simulink model "wb_poco_al_intfract_v00"  (Simulink 6.2)
settings: Solver=ode45  StartTime=0.0  StopTime=2^23  RelTol=1e-3
libraries: xbsIndex_r3 x705, xps_library x24, delay_lib x6, fft_library x2, pfb_library x1
(part 1 of 6)
settings Model: LastModifiedBy=sandeep
settings DebuggingCC: SolverPrmCheckMsg=warning

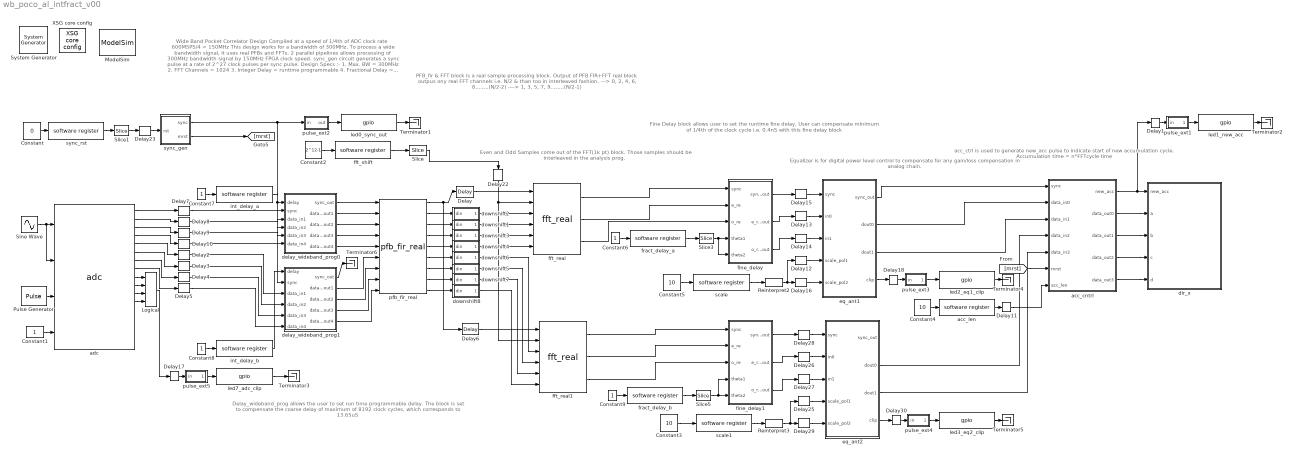
== system wb_poco_al_intfract_v00 ==
  note: Even and Odd Samples come out of the FFT(1k pt) block.
      | Those samples should be interleaved in the analysis prog.
  note: Wide Band Pocket Correlator Design Compiled at a speed of 1/4th of ADC clock rate 600MSPS/4 = 150MHz
      | This design works for a bandwidth of 300MHz. To process a wide bandwidth signal, it uses real PFBs and FFTs.
      | 2 parallel pipelines allows processing of 300MHz bandwidth signal by 150MHz FPGA clock speed.
      | sync_gen circuit generates a sync pulse at a rate of 2^27 clock pulses per sync pulse.
      | Design Specs :-
      | 1. Max. BW = 300MHz
      | 2. FFT Channels = 1024
      | 3. Integer Delay = runtime programmable
      | 4. Fractional Delay = runtime programmable
      | 5. Accumulation time = user cofigurable
  note: PFB_fir & FFT block is a real sample processing block.
      | Output of PFB FIR+FFT real block outpus ony real FFT channels i.e. N/2
      | & than too in interleaved fashion.
      | ---> 0, 2, 4, 6, 8........(N/2-2)
      | ----> 1, 3, 5, 7, 9........(N/2-1)
  note: Equalizer is for digital power level control
      | to compensate for any gain/loss compensation in analog chain.
  note: acc_ctrl is used to generate new_acc pulse
      | to indicate start of new accumulation cycle.
      | Accumulation time = n*FFTcycle time
  note: Delay_wideband_prog allows the user to set run time programmable delay.
      | The block is set to compensate the coarse delay of  maximum of 8192 clock cycles,
      | which corresponds to 13.65uS
  note: Fine Delay block allows user to set the runtime fine delay.
      | User can compensate minimum of 1/4th of the clock cycle i.e. 0.4nS with this fine delay block
  " System Generator" : xbsIndex_r3/ System Generator  Tag=genX  xilinxfamily=Virtex2P  part=xc2vp50  speed=-7  package=ff1152  synthesis_tool=XST  directory=./wb_poco_al_intfract_v00/sysgen  testbench=off  simulink_period=1  sysclk_period=6.6225  incr_netlist=off  trim_vbits=Everywhere in SubSystem  dbl_ovrd=According to Block Masks  core_generation=According to Block Masks  run_coregen=off  deprecated_control=off  eval_field=0
      settings: AttributesFormatString=System\nGenerator
  Constant : Constant  Value=0
  Constant{1,6..9} (5 alike) : Constant
  Constant2 : Constant  Value=2^12-1
  Constant3 : Constant  Value=10
  Constant4 : Constant  Value=10
  Constant5 : Constant  Value=10
  Delay : xbsIndex_r3/Delay  latency=2  reg_retiming=off  explicit_period=off  period=1  en=off  accept_only_valid=off  init_zero=on  dbl_ovrd=off  show_param=off
      settings: xl_area=[0, 0, 0, 0, 0, 0, 0]
  Delay{1,11..18,23,25..30} (16 alike) : xbsIndex_r3/Delay  latency=3  reg_retiming=on  explicit_period=off  period=1  en=off  accept_only_valid=off  init_zero=on  dbl_ovrd=off  show_param=off
      settings: xl_area=[0, 0, 0, 0, 0, 0, 0]
  Delay{2..5,7..10} (8 alike) : xbsIndex_r3/Delay  latency=2  reg_retiming=on  explicit_period=off  period=1  en=off  accept_only_valid=off  init_zero=on  dbl_ovrd=off  show_param=off
      settings: xl_area=[0, 0, 0, 0, 0, 0, 0]
  Delay22 : xbsIndex_r3/Delay  Orientation=down  latency=5  reg_retiming=on  explicit_period=off  period=1  en=off  accept_only_valid=off  init_zero=on  dbl_ovrd=off  show_param=off
      settings: xl_area=[0, 0, 0, 0, 0, 0, 0]
  Delay6 : xbsIndex_r3/Delay  latency=2  reg_retiming=off  explicit_period=off  period=1  en=off  accept_only_valid=off  init_zero=on  dbl_ovrd=off  show_param=off
      settings: xl_area=[0, 0, 0, 0, 0, 0, 0]
  Logical : xbsIndex_r3/Logical  logical_function=OR  inputs=4  precision=Full  arith_type=Unsigned  n_bits=8  bin_pt=2  align_bp=on  latency=0  explicit_period=off  period=1  en=off  dbl_ovrd=off  show_param=off
      settings: xl_area=[0, 0, 0, 0, 0, 0, 0]
  ModelSim : xbsIndex_r3/ModelSim  dir=./modelsim  waveform=on  leave_open=on  skip_compile=off  custom_scripts=off  startup_timeout=40
  Pulse Generator : DiscretePulseGenerator  Period=2^27
  Reinterpret2 : xbsIndex_r3/Reinterpret  force_arith_type=on  arith_type=Unsigned  force_bin_pt=on  bin_pt=3  force_valid=on
  Reinterpret3 : xbsIndex_r3/Reinterpret  force_arith_type=on  arith_type=Unsigned  force_bin_pt=on  bin_pt=3  force_valid=on
  Sine Wave : Sin  SineType=Sample based  Frequency=1/4  Samples=16  SampleTime=0.25
  Slice : xbsIndex_r3/Slice  mode=Upper Bit Location + Width  nbits=12  bit1=0  base1=MSB of Input  bit0=0  base0=LSB of Input  boolean_output=off  explicit_period=off  period=1  dbl_ovrd=off
  Slice1 : xbsIndex_r3/Slice  mode=Lower Bit Location + Width  nbits=1  bit1=0  base1=MSB of Input  bit0=0  base0=LSB of Input  boolean_output=on  explicit_period=off  period=1  dbl_ovrd=off
  Slice3 : xbsIndex_r3/Slice  mode=Lower Bit Location + Width  nbits=8  bit1=0  base1=MSB of Input  bit0=0  base0=LSB of Input  boolean_output=off  explicit_period=off  period=1  dbl_ovrd=off
  Slice5 : xbsIndex_r3/Slice  mode=Lower Bit Location + Width  nbits=8  bit1=0  base1=MSB of Input  bit0=0  base0=LSB of Input  boolean_output=off  explicit_period=off  period=1  dbl_ovrd=off
  Terminator{1..6} (6 alike) : Terminator
  XSG core config : xps_library/XSG core config  Tag=xps:xsg  hw_sys=iBOB  ibob_linux=off  clk_src=adc1_clk  gpio_clk_io_group=iBOB:sma  gpio_clk_bit_index=0  clk_rate=151  sample_period=1  synthesis_tool=XST  mpc_type=powerpc405
  acc_cntrl : Subsystem  mask{chan_bits=8}
      mask prompts: chan_bits "Number of Channels (2^?)"
  acc_len : xps_library/software register  Tag=xps:sw_reg  io_dir=From Processor  arith_type=Unsigned  bitwidth=32  bin_pt=0  sample_period=1  gw_name=wb_poco_al_intfract_v00_acc_len_user_data_out
  adc : xps_library/adc  Tag=xps:adc  adc_brd=iBOB:adc1  adc_clk_rate=601  adc_interleave=off  sample_period=1
  delay_wideband_prog0 : Subsystem
      settings: AttributesFormatString=Min Delay=28
  delay_wideband_prog1 : Subsystem
      settings: AttributesFormatString=Min Delay=28
  dir_x : Subsystem  mask{n_chans=1024}
      mask prompts: n_chans "Number of Channels"
  downshift1 : Subsystem
  downshift2 : Subsystem
  downshift3 : Subsystem
  downshift4 : Subsystem
  downshift5 : Subsystem
  downshift6 : Subsystem
  downshift7 : Subsystem
  downshift8 : Subsystem
  eq_ant1 : Subsystem  mask{n_chans=512}
      mask prompts: n_chans "Number of Channels"
      mask init:
      | chan_bits=ceil(log2(n_chans));
  eq_ant2 : Subsystem  mask{n_chans=512}
      mask prompts: n_chans "Number of Channels"
      mask init:
      | chan_bits=ceil(log2(n_chans));
  fft_real : fft_library/fft_real  FFTSize=10  BitWidth=18  n_inputs=2  quantization="Round  (unbiased: Even Values)"  overflow=Wrap  add_latency=2  mult_latency=3  bram_latency=2
  fft_real1 : fft_library/fft_real  FFTSize=10  BitWidth=18  n_inputs=2  quantization="Round  (unbiased: Even Values)"  overflow=Wrap  add_latency=2  mult_latency=3  bram_latency=2
  fft_shift : xps_library/software register  Tag=xps:sw_reg  io_dir=From Processor  arith_type=Unsigned  bitwidth=32  bin_pt=0  sample_period=1  gw_name=wb_poco_al_intfract_v00_fft_shift_user_data_out
  fine_delay : Subsystem  AncestorBlock=delay_lib/fine_delay  mask{fft_len=1024, fft_bits=18, theta_bits=11, sine_cos_bits=18}
      mask prompts: fft_len "Number Of FFT Channels"; fft_bits "FFT Input Bit Width"; theta_bits "Sine-Cos LUT Input Bitwidth (Determines the resolution of phase)"; sine_cos_bits "Sine-Cos LUT Output Data Width"
      mask init:
      | %fine_delay_init(gcb,...
      |  %   'fft_len',fft_len,...
      |   %  'fft_bits',fft_bits...
      |    % 'theta_bits',theta_bits,...
      |     %'sine_cos_bits',sine_cos_bits)
  fine_delay1 : Subsystem  AncestorBlock=delay_lib/fine_delay  mask{fft_len=1024, fft_bits=18, theta_bits=11, sine_cos_bits=18}
      mask prompts: fft_len "Number Of FFT Channels"; fft_bits "FFT Input Bit Width"; theta_bits "Sine-Cos LUT Input Bitwidth (Determines the resolution of phase)"; sine_cos_bits "Sine-Cos LUT Output Data Width"
      mask init:
      | %fine_delay_init(gcb,...
      |  %   'fft_len',fft_len,...
      |   %  'fft_bits',fft_bits...
      |    % 'theta_bits',theta_bits,...
      |     %'sine_cos_bits',sine_cos_bits)
  fract_delay_a : xps_library/software register  Tag=xps:sw_reg  io_dir=From Processor  arith_type=Unsigned  bitwidth=32  bin_pt=0  sample_period=1  gw_name=wb_poco_al_intfract_v00_fract_delay_a_user_data_out
  fract_delay_b : xps_library/software register  Tag=xps:sw_reg  io_dir=From Processor  arith_type=Unsigned  bitwidth=32  bin_pt=0  sample_period=1  gw_name=wb_poco_al_intfract_v00_fract_delay_b_user_data_out
  int_delay_a : xps_library/software register  Tag=xps:sw_reg  io_dir=From Processor  arith_type=Unsigned  bitwidth=32  bin_pt=0  sample_period=1  gw_name=wb_poco_al_intfract_v00_int_delay_a_user_data_out
  int_delay_b : xps_library/software register  Tag=xps:sw_reg  io_dir=From Processor  arith_type=Unsigned  bitwidth=32  bin_pt=0  sample_period=1  gw_name=wb_poco_al_intfract_v00_int_delay_b_user_data_out
  led0_sync_out : xps_library/gpio  Tag=xps:gpio  io_group=iBOB:led  io_dir=out  arith_type=Boolean  bitwidth=1  bin_pt=0  bit_index=0  sample_period=1  use_single_ended=off  use_ddr=off  reg_iob=on  reg_clk_phase=0  termination=None
  led1_new_acc : xps_library/gpio  Tag=xps:gpio  io_group=iBOB:led  io_dir=out  arith_type=Boolean  bitwidth=1  bin_pt=0  bit_index=1  sample_period=1  use_single_ended=off  use_ddr=off  reg_iob=on  reg_clk_phase=0  termination=None
  led2_eq1_clip : xps_library/gpio  Tag=xps:gpio  io_group=iBOB:led  io_dir=out  arith_type=Boolean  bitwidth=1  bin_pt=0  bit_index=2  sample_period=1  use_single_ended=off  use_ddr=off  reg_iob=on  reg_clk_phase=0  termination=None
  led3_eq2_clip : xps_library/gpio  Tag=xps:gpio  io_group=iBOB:led  io_dir=out  arith_type=Boolean  bitwidth=1  bin_pt=0  bit_index=3  sample_period=1  use_single_ended=off  use_ddr=off  reg_iob=on  reg_clk_phase=0  termination=None
  led7_adc_clip : xps_library/gpio  Tag=xps:gpio  io_group=iBOB:led  io_dir=out  arith_type=Boolean  bitwidth=1  bin_pt=0  bit_index=7  sample_period=1  use_single_ended=off  use_ddr=off  reg_iob=on  reg_clk_phase=0  termination=None
  pfb_fir_real : pfb_library/pfb_fir_real  PFBSize=10  TotalTaps=4  WindowType=hamming  n_inputs=2  MakeBiplex=on  BitWidthIn=8  BitWidthOut=18  CoeffBitWidth=8  CoeffDistMem=off  add_latency=2  mult_latency=3  bram_latency=2  quantization="Round  (unbiased: +/- Inf)"  fwidth=1
      link override pol1_in1_first_tap/sync_delay/Constant: equ=P=C
      link override pol1_in1_first_tap/sync_delay/Constant1: equ=P=C
      link override pol1_in1_first_tap/sync_delay/Constant2: equ=P=C
      link override pol1_in1_first_tap/sync_delay/Constant3: equ=P=C
      link override pol1_in1_tap2/sync_delay/Constant: equ=P=C
      link override pol1_in1_tap2/sync_delay/Constant1: equ=P=C
      link override pol1_in1_tap2/sync_delay/Constant2: equ=P=C
      link override pol1_in1_tap2/sync_delay/Constant3: equ=P=C
      link override pol1_in1_tap3/sync_delay/Constant: equ=P=C
      link override pol1_in1_tap3/sync_delay/Constant1: equ=P=C
      link override pol1_in1_tap3/sync_delay/Constant2: equ=P=C
      link override pol1_in1_tap3/sync_delay/Constant3: equ=P=C
      link override pol1_in2_first_tap/sync_delay/Constant: equ=P=C
      link override pol1_in2_first_tap/sync_delay/Constant1: equ=P=C
      link override pol1_in2_first_tap/sync_delay/Constant2: equ=P=C
      link override pol1_in2_first_tap/sync_delay/Constant3: equ=P=C
      link override pol1_in2_tap2/sync_delay/Constant: equ=P=C
      link override pol1_in2_tap2/sync_delay/Constant1: equ=P=C
      link override pol1_in2_tap2/sync_delay/Constant2: equ=P=C
      link override pol1_in2_tap2/sync_delay/Constant3: equ=P=C
      link override pol1_in2_tap3/sync_delay/Constant: equ=P=C
      link override pol1_in2_tap3/sync_delay/Constant1: equ=P=C
      link override pol1_in2_tap3/sync_delay/Constant2: equ=P=C
      link override pol1_in2_tap3/sync_delay/Constant3: equ=P=C
      link override pol1_in3_first_tap/sync_delay/Constant: equ=P=C
      link override pol1_in3_first_tap/sync_delay/Constant1: equ=P=C
      link override pol1_in3_first_tap/sync_delay/Constant2: equ=P=C
      link override pol1_in3_first_tap/sync_delay/Constant3: equ=P=C
      link override pol1_in3_tap2/sync_delay/Constant: equ=P=C
      link override pol1_in3_tap2/sync_delay/Constant1: equ=P=C
      link override pol1_in3_tap2/sync_delay/Constant2: equ=P=C
      link override pol1_in3_tap2/sync_delay/Constant3: equ=P=C
      link override pol1_in3_tap3/sync_delay/Constant: equ=P=C
      link override pol1_in3_tap3/sync_delay/Constant1: equ=P=C
      link override pol1_in3_tap3/sync_delay/Constant2: equ=P=C
      link override pol1_in3_tap3/sync_delay/Constant3: equ=P=C
      link override pol1_in4_first_tap/sync_delay/Constant: equ=P=C
      link override pol1_in4_first_tap/sync_delay/Constant1: equ=P=C
      link override pol1_in4_first_tap/sync_delay/Constant2: equ=P=C
      link override pol1_in4_first_tap/sync_delay/Constant3: equ=P=C
      link override pol1_in4_tap2/sync_delay/Constant: equ=P=C
      link override pol1_in4_tap2/sync_delay/Constant1: equ=P=C
      link override pol1_in4_tap2/sync_delay/Constant2: equ=P=C
      link override pol1_in4_tap2/sync_delay/Constant3: equ=P=C
      link override pol1_in4_tap3/sync_delay/Constant: equ=P=C
      link override pol1_in4_tap3/sync_delay/Constant1: equ=P=C
      link override pol1_in4_tap3/sync_delay/Constant2: equ=P=C
      link override pol1_in4_tap3/sync_delay/Constant3: equ=P=C
      link override pol2_in1_first_tap/sync_delay/Constant: equ=P=C
      link override pol2_in1_first_tap/sync_delay/Constant1: equ=P=C
      link override pol2_in1_first_tap/sync_delay/Constant2: equ=P=C
      link override pol2_in1_first_tap/sync_delay/Constant3: equ=P=C
      link override pol2_in1_tap2/sync_delay/Constant: equ=P=C
      link override pol2_in1_tap2/sync_delay/Constant1: equ=P=C
      link override pol2_in1_tap2/sync_delay/Constant2: equ=P=C
      link override pol2_in1_tap2/sync_delay/Constant3: equ=P=C
      link override pol2_in1_tap3/sync_delay/Constant: equ=P=C
      link override pol2_in1_tap3/sync_delay/Constant1: equ=P=C
      link override pol2_in1_tap3/sync_delay/Constant2: equ=P=C
      link override pol2_in1_tap3/sync_delay/Constant3: equ=P=C
      link override pol2_in2_first_tap/sync_delay/Constant: equ=P=C
      link override pol2_in2_first_tap/sync_delay/Constant1: equ=P=C
      link override pol2_in2_first_tap/sync_delay/Constant2: equ=P=C
      link override pol2_in2_first_tap/sync_delay/Constant3: equ=P=C
      link override pol2_in2_tap2/sync_delay/Constant: equ=P=C
      link override pol2_in2_tap2/sync_delay/Constant1: equ=P=C
      link override pol2_in2_tap2/sync_delay/Constant2: equ=P=C
      link override pol2_in2_tap2/sync_delay/Constant3: equ=P=C
      link override pol2_in2_tap3/sync_delay/Constant: equ=P=C
      link override pol2_in2_tap3/sync_delay/Constant1: equ=P=C
      link override pol2_in2_tap3/sync_delay/Constant2: equ=P=C
      link override pol2_in2_tap3/sync_delay/Constant3: equ=P=C
      link override pol2_in3_first_tap/sync_delay/Constant: equ=P=C
      link override pol2_in3_first_tap/sync_delay/Constant1: equ=P=C
      link override pol2_in3_first_tap/sync_delay/Constant2: equ=P=C
      link override pol2_in3_first_tap/sync_delay/Constant3: equ=P=C
      link override pol2_in3_tap2/sync_delay/Constant: equ=P=C
      link override pol2_in3_tap2/sync_delay/Constant1: equ=P=C
      link override pol2_in3_tap2/sync_delay/Constant2: equ=P=C
      link override pol2_in3_tap2/sync_delay/Constant3: equ=P=C
      link override pol2_in3_tap3/sync_delay/Constant: equ=P=C
      link override pol2_in3_tap3/sync_delay/Constant1: equ=P=C
      link override pol2_in3_tap3/sync_delay/Constant2: equ=P=C
      link override pol2_in3_tap3/sync_delay/Constant3: equ=P=C
      link override pol2_in4_first_tap/sync_delay/Constant: equ=P=C
      link override pol2_in4_first_tap/sync_delay/Constant1: equ=P=C
      link override pol2_in4_first_tap/sync_delay/Constant2: equ=P=C
      link override pol2_in4_first_tap/sync_delay/Constant3: equ=P=C
      link override pol2_in4_tap2/sync_delay/Constant: equ=P=C
      link override pol2_in4_tap2/sync_delay/Constant1: equ=P=C
      link override pol2_in4_tap2/sync_delay/Constant2: equ=P=C
      link override pol2_in4_tap2/sync_delay/Constant3: equ=P=C
      link override pol2_in4_tap3/sync_delay/Constant: equ=P=C
      link override pol2_in4_tap3/sync_delay/Constant1: equ=P=C
      link override pol2_in4_tap3/sync_delay/Constant2: equ=P=C
      link override pol2_in4_tap3/sync_delay/Constant3: equ=P=C
  pulse_ext1 : Subsystem  mask{pulse_len=2^23}
      mask prompts: pulse_len "Length of Pulse"
      mask init:
      | bits = ceil(log2(pulse_len+1));
  pulse_ext2 : Subsystem  mask{pulse_len=2^23}
      mask prompts: pulse_len "Length of Pulse"
      mask init:
      | bits = ceil(log2(pulse_len+1));
  pulse_ext3 : Subsystem  mask{pulse_len=2^23}
      mask prompts: pulse_len "Length of Pulse"
      mask init:
      | bits = ceil(log2(pulse_len+1));
  pulse_ext4 : Subsystem  mask{pulse_len=2^23}
      mask prompts: pulse_len "Length of Pulse"
      mask init:
      | bits = ceil(log2(pulse_len+1));
  pulse_ext5 : Subsystem  mask{pulse_len=2^23}
      mask prompts: pulse_len "Length of Pulse"
      mask init:
      | bits = ceil(log2(pulse_len+1));
  scale : xps_library/software register  Tag=xps:sw_reg  io_dir=From Processor  arith_type=Unsigned  bitwidth=32  bin_pt=0  sample_period=1  gw_name=wb_poco_al_intfract_v00_scale_user_data_out
  scale1 : xps_library/software register  Tag=xps:sw_reg  io_dir=From Processor  arith_type=Unsigned  bitwidth=32  bin_pt=0  sample_period=1  gw_name=wb_poco_al_intfract_v00_scale1_user_data_out
  sync_gen : Subsystem  mask{sync_bits=27}
      mask prompts: sync_bits "Sync Period (2^?)"
  sync_rst : xps_library/software register  Tag=xps:sw_reg  io_dir=From Processor  arith_type=Unsigned  bitwidth=32  bin_pt=0  sample_period=1  gw_name=wb_poco_al_intfract_v00_sync_rst_user_data_out
  wires:
  Sine Wave/1 -> adc/1, adc/2
  sync_gen/1(sync) -> pulse_ext2/1(in), delay_wideband_prog0/2(sync), delay_wideband_prog1/2(sync)
  sync_gen/2(mrst) -> [mrst]
  Constant/1 -> sync_rst/1
  sync_rst/1 -> Slice1/1
  Slice1/1 -> Delay23/1
  led0_sync_out/1 -> Terminator1/1
  Pulse Generator/1 -> adc/3
  Constant1/1 -> adc/4
  adc/1 -> Delay7/1
  adc/2 -> Delay8/1
  adc/3 -> Delay9/1
  adc/4 -> Delay10/1
  pfb_fir_real/1 -> Delay/1, Delay6/1
  Constant2/1 -> fft_shift/1
  fft_shift/1 -> Slice/1
  Delay/1 -> fft_real/1
  pfb_fir_real/2 -> downshift2/1(din)
  pfb_fir_real/3 -> downshift1/1(din)
  pfb_fir_real/4 -> downshift3/1(din)
  pfb_fir_real/5 -> downshift4/1(din)
  Slice/1 -> Delay22/1
  downshift2/1(dout) -> fft_real/3
  downshift1/1(dout) -> fft_real/4
  downshift3/1(dout) -> fft_real/5
  downshift4/1(dout) -> fft_real/6
  Delay13/1 -> eq_ant1/2(in0)
  Delay14/1 -> eq_ant1/3(in1)
  Delay15/1 -> eq_ant1/1(sync)
  pulse_ext2/1(out) -> led0_sync_out/1
  pulse_ext3/1(out) -> led2_eq1_clip/1
  eq_ant1/4(clip) -> Delay18/1
  Constant5/1 -> scale/1
  scale/1 -> Reinterpret2/1
  Delay12/1 -> eq_ant1/4(scale_pol1)
  Delay16/1 -> eq_ant1/5(scale_pol2)
  Delay18/1 -> pulse_ext3/1(in)
  Delay22/1 -> fft_real/2, fft_real1/2
  Delay23/1 -> sync_gen/1(rst)
  Reinterpret2/1 -> Delay12/1, Delay16/1
  adc/5 -> Delay2/1
  adc/6 -> Delay3/1
  adc/7 -> Delay4/1
  adc/8 -> Delay5/1
  Delay6/1 -> fft_real1/1
  downshift6/1(dout) -> fft_real1/3
  downshift5/1(dout) -> fft_real1/4
  downshift7/1(dout) -> fft_real1/5
  downshift8/1(dout) -> fft_real1/6
  pfb_fir_real/6 -> downshift6/1(din)
  pfb_fir_real/7 -> downshift5/1(din)
  pfb_fir_real/8 -> downshift7/1(din)
  pfb_fir_real/9 -> downshift8/1(din)
  Delay26/1 -> eq_ant2/2(in0)
  Delay27/1 -> eq_ant2/3(in1)
  Delay28/1 -> eq_ant2/1(sync)
  pulse_ext4/1(out) -> led3_eq2_clip/1
  eq_ant2/4(clip) -> Delay30/1
  Delay25/1 -> eq_ant2/4(scale_pol1)
  Delay29/1 -> eq_ant2/5(scale_pol2)
  Delay30/1 -> pulse_ext4/1(in)
  Constant3/1 -> scale1/1
  scale1/1 -> Reinterpret3/1
  Reinterpret3/1 -> Delay29/1, Delay25/1
  led2_eq1_clip/1 -> Terminator4/1
  led3_eq2_clip/1 -> Terminator5/1
  Constant4/1 -> acc_len/1
  acc_len/1 -> Delay11/1
  Delay11/1 -> acc_cntrl/7(acc_len)
  [mrst] -> acc_cntrl/6(mrst)
  eq_ant1/1(sync_out) -> acc_cntrl/1(sync)
  eq_ant1/2(dout0) -> acc_cntrl/2(data_in0)
  eq_ant1/3(dout1) -> acc_cntrl/3(data_in1)
  eq_ant2/2(dout0) -> acc_cntrl/4(data_in2)
  eq_ant2/3(dout1) -> acc_cntrl/5(data_in3)
  acc_cntrl/1(new_acc) -> dir_x/1(new_acc), Delay1/1
  acc_cntrl/2(data_out0) -> dir_x/2(a)
  acc_cntrl/3(data_out1) -> dir_x/3(b)
  acc_cntrl/4(data_out2) -> dir_x/4(c)
  acc_cntrl/5(data_out3) -> dir_x/5(d)
  pulse_ext1/1(out) -> led1_new_acc/1
  Delay1/1 -> pulse_ext1/1(in)
  led1_new_acc/1 -> Terminator2/1
  pulse_ext5/1(out) -> led7_adc_clip/1
  Delay17/1 -> pulse_ext5/1(in)
  led7_adc_clip/1 -> Terminator3/1
  adc/9 -> Logical/1
  adc/10 -> Logical/2
  adc/11 -> Logical/3
  adc/12 -> Logical/4
  Logical/1 -> Delay17/1
  int_delay_a/1 -> delay_wideband_prog0/1(delay)
  int_delay_b/1 -> delay_wideband_prog1/1(delay)
  Constant7/1 -> int_delay_a/1
  Constant8/1 -> int_delay_b/1
  delay_wideband_prog0/1(sync_out) -> pfb_fir_real/1
  delay_wideband_prog0/2(data_out1) -> pfb_fir_real/2
  delay_wideband_prog0/3(data_out2) -> pfb_fir_real/3
  delay_wideband_prog0/4(data_out3) -> pfb_fir_real/4
  delay_wideband_prog0/5(data_out4) -> pfb_fir_real/5
  Delay7/1 -> delay_wideband_prog0/3(data_in1)
  Delay8/1 -> delay_wideband_prog0/4(data_in2)
  Delay9/1 -> delay_wideband_prog0/5(data_in3)
  Delay10/1 -> delay_wideband_prog0/6(data_in4)
  delay_wideband_prog1/1(sync_out) -> Terminator6/1
  Delay2/1 -> delay_wideband_prog1/3(data_in1)
  Delay3/1 -> delay_wideband_prog1/4(data_in2)
  Delay4/1 -> delay_wideband_prog1/5(data_in3)
  Delay5/1 -> delay_wideband_prog1/6(data_in4)
  delay_wideband_prog1/2(data_out1) -> pfb_fir_real/6
  delay_wideband_prog1/3(data_out2) -> pfb_fir_real/7
  delay_wideband_prog1/4(data_out3) -> pfb_fir_real/8
  delay_wideband_prog1/5(data_out4) -> pfb_fir_real/9
  Constant6/1 -> fract_delay_a/1
  fract_delay_a/1 -> Slice3/1
  Slice3/1 -> fine_delay/4(theta1), fine_delay/5(theta2)
  fft_real/1 -> fine_delay/1(sync)
  fft_real/2 -> fine_delay/2(e_re)
  fft_real/3 -> fine_delay/3(o_re)
  Constant9/1 -> fract_delay_b/1
  fract_delay_b/1 -> Slice5/1
  fine_delay/1(sync_out) -> Delay15/1
  fine_delay/2(e_re_out) -> Delay13/1
  fine_delay/3(o_re_out) -> Delay14/1
  fine_delay1/1(sync_out) -> Delay28/1
  fine_delay1/2(e_re_out) -> Delay26/1
  fine_delay1/3(o_re_out) -> Delay27/1
  Slice5/1 -> fine_delay1/5(theta2), fine_delay1/4(theta1)
  fft_real1/1 -> fine_delay1/1(sync)
  fft_real1/2 -> fine_delay1/2(e_re)
  fft_real1/3 -> fine_delay1/3(o_re)

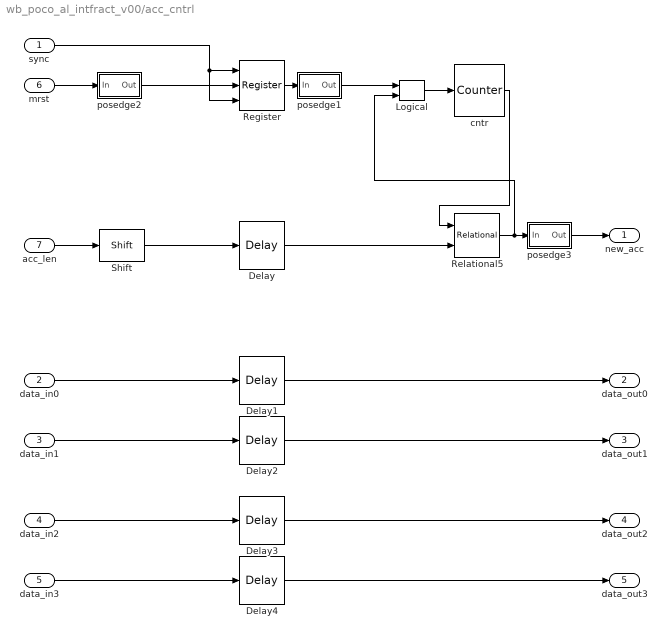
== system wb_poco_al_intfract_v00/acc_cntrl ==
  sync : Inport  Port=1  LatchInput=off
  data_in0 : Inport  Port=2  LatchInput=off
  data_in1 : Inport  Port=3  LatchInput=off
  data_in2 : Inport  Port=4  LatchInput=off
  data_in3 : Inport  Port=5  LatchInput=off
  mrst : Inport  Port=6  LatchInput=off
  acc_len : Inport  Port=7  LatchInput=off
  Delay{,1..4} (5 alike) : xbsIndex_r3/Delay  latency=1  reg_retiming=on  explicit_period=off  period=1  en=off  accept_only_valid=off  init_zero=on  dbl_ovrd=off  show_param=off
      settings: xl_area=[0, 0, 0, 0, 0, 0, 0]
  Logical : xbsIndex_r3/Logical  logical_function=OR  inputs=2  precision=Full  arith_type=Unsigned  n_bits=8  bin_pt=2  align_bp=on  latency=0  explicit_period=off  period=1  en=off  dbl_ovrd=off  show_param=off
      settings: xl_area=[0, 0, 0, 0, 0, 0, 0]
  Register : xbsIndex_r3/Register  init=0  reg_only_valid=off  explicit_period=off  period=1  rst=on  en=on  out_en=off  dbl_ovrd=off  show_param=off
      settings: xl_area=[0, 0, 0, 0, 0, 0, 0]
  Relational5 : xbsIndex_r3/Relational  mode=a>=b  latency=0  explicit_period=on  period=1  en=off  dbl_ovrd=off  show_param=off
      settings: xl_area=[0, 0, 0, 0, 0, 0, 0]
  Shift : xbsIndex_r3/Shift  shift_dir=Left  shift_bits=chan_bits  precision=Full  arith_type="Signed  (2's comp)"  n_bits=8  bin_pt=2  quantization=Truncate  overflow=Wrap  latency=0  explicit_period=off  period=1  en=off  dbl_ovrd=off  show_param=off
      settings: xl_area=[0, 0, 0, 0, 0, 0, 0]
  cntr : xbsIndex_r3/Counter  cnt_type=Free Running  n_bits=32  bin_pt=0  arith_type=Unsigned  start_count=1  cnt_to=Inf  cnt_by_val=1  operation=Up  explicit_period=on  period=1  load_pin=off  rst=on  en=off  dbl_ovrd=off  show_param=off  use_rpm=on  gen_core=off
      settings: xl_area=[0, 0, 0, 0, 0, 0, 0]
  posedge1 : Subsystem  Tag=Rising Edge Detector
  posedge2 : Subsystem  Tag=Rising Edge Detector
  posedge3 : Subsystem  Tag=Rising Edge Detector
  new_acc : Outport
  data_out0 : Outport  Port=2
  data_out1 : Outport  Port=3
  data_out2 : Outport  Port=4
  data_out3 : Outport  Port=5
  wires:
  Relational5/1 -> Logical/2, posedge3/1(In)
  acc_len/1 -> Shift/1
  data_in0/1 -> Delay1/1
  posedge3/1(Out) -> new_acc/1
  Logical/1 -> cntr/1
  Register/1 -> posedge1/1(In)
  posedge2/1(Out) -> Register/2
  posedge1/1(Out) -> Logical/1
  Delay/1 -> Relational5/2
  Delay1/1 -> data_out0/1
  Shift/1 -> Delay/1
  cntr/1 -> Relational5/1
  mrst/1 -> posedge2/1(In)
  sync/1 -> Register/1, Register/3
  data_in1/1 -> Delay2/1
  Delay2/1 -> data_out1/1
  data_in2/1 -> Delay3/1
  Delay3/1 -> data_out2/1
  data_in3/1 -> Delay4/1
  Delay4/1 -> data_out3/1

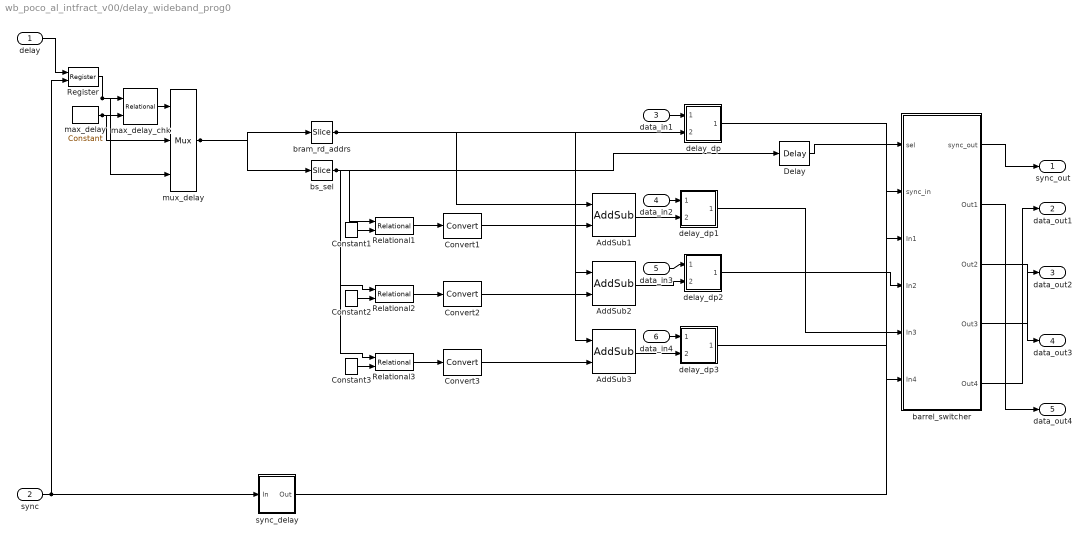
== system wb_poco_al_intfract_v00/delay_wideband_prog0 ==
  delay : Inport  Port=1  LatchInput=off
  sync : Inport  Port=2  LatchInput=off
  data_in1 : Inport  Port=3  LatchInput=off
  data_in2 : Inport  Port=4  LatchInput=off
  data_in3 : Inport  Port=5  LatchInput=off
  data_in4 : Inport  Port=6  LatchInput=off
  AddSub1 : xbsIndex_r3/AddSub  mode=Addition  precision=Full  arith_type=Unsigned  n_bits=11  bin_pt=0  quantization=Truncate  overflow=Wrap  latency=0  explicit_period=off  period=1  use_carryin=off  use_carryout=off  en=off  dbl_ovrd=off  show_param=off  use_core=on  pipeline=off  use_rpm=on  gen_core=off
      settings: xl_area=[0, 0, 0, 0, 0, 0, 0]
  AddSub2 : xbsIndex_r3/AddSub  mode=Addition  precision=Full  arith_type=Unsigned  n_bits=11  bin_pt=0  quantization=Truncate  overflow=Wrap  latency=0  explicit_period=off  period=1  use_carryin=off  use_carryout=off  en=off  dbl_ovrd=off  show_param=off  use_core=on  pipeline=off  use_rpm=on  gen_core=off
      settings: xl_area=[0, 0, 0, 0, 0, 0, 0]
  AddSub3 : xbsIndex_r3/AddSub  mode=Addition  precision=Full  arith_type=Unsigned  n_bits=11  bin_pt=0  quantization=Truncate  overflow=Wrap  latency=0  explicit_period=off  period=1  use_carryin=off  use_carryout=off  en=off  dbl_ovrd=off  show_param=off  use_core=on  pipeline=off  use_rpm=on  gen_core=off
      settings: xl_area=[0, 0, 0, 0, 0, 0, 0]
  Constant1 : xbsIndex_r3/Constant  const=2  equ=P=C  arith_type=Unsigned  n_bits=2  bin_pt=0  opselect=C  inp2=PCIN>>17  opr=+  inp1=P  carry=CIN  iostate=0  explicit_period=on  period=1  dbl_ovrd=off
  Constant2 : xbsIndex_r3/Constant  const=1  equ=P=C  arith_type=Unsigned  n_bits=2  bin_pt=0  opselect=C  inp2=PCIN>>17  opr=+  inp1=P  carry=CIN  iostate=0  explicit_period=on  period=1  dbl_ovrd=off
  Constant3 : xbsIndex_r3/Constant  const=0  equ=P=C  arith_type=Unsigned  n_bits=2  bin_pt=0  opselect=C  inp2=PCIN>>17  opr=+  inp1=P  carry=CIN  iostate=0  explicit_period=on  period=1  dbl_ovrd=off
  Convert1 : xbsIndex_r3/Convert  arith_type=Unsigned  n_bits=1  bin_pt=0  quantization=Truncate  overflow=Wrap  latency=0  explicit_period=off  period=1  dbl_ovrd=off  show_param=off  inserted_by_tool=off  pipeline=off
      settings: xl_area=[0, 0, 0, 0, 0, 0, 0]
  Convert2 : xbsIndex_r3/Convert  arith_type=Unsigned  n_bits=1  bin_pt=0  quantization=Truncate  overflow=Wrap  latency=0  explicit_period=off  period=1  dbl_ovrd=off  show_param=off  inserted_by_tool=off  pipeline=off
      settings: xl_area=[0, 0, 0, 0, 0, 0, 0]
  Convert3 : xbsIndex_r3/Convert  arith_type=Unsigned  n_bits=1  bin_pt=0  quantization=Truncate  overflow=Wrap  latency=0  explicit_period=off  period=1  dbl_ovrd=off  show_param=off  inserted_by_tool=off  pipeline=off
      settings: xl_area=[0, 0, 0, 0, 0, 0, 0]
  Delay : xbsIndex_r3/Delay  latency=5  reg_retiming=off  explicit_period=off  period=1  en=off  accept_only_valid=off  init_zero=on  dbl_ovrd=off  show_param=off
      settings: xl_area=[0, 0, 0, 0, 0, 0, 0]
  Register : xbsIndex_r3/Register  init=0  reg_only_valid=off  explicit_period=off  period=1  rst=off  en=on  out_en=off  dbl_ovrd=off  show_param=off
      settings: xl_area=[0, 0, 0, 0, 0, 0, 0]
  Relational1 : xbsIndex_r3/Relational  mode=a>b  latency=0  explicit_period=off  period=1  en=off  dbl_ovrd=off  show_param=off
      settings: xl_area=[0, 0, 0, 0, 0, 0, 0]
  Relational2 : xbsIndex_r3/Relational  mode=a>b  latency=0  explicit_period=off  period=1  en=off  dbl_ovrd=off  show_param=off
      settings: xl_area=[0, 0, 0, 0, 0, 0, 0]
  Relational3 : xbsIndex_r3/Relational  mode=a>b  latency=0  explicit_period=off  period=1  en=off  dbl_ovrd=off  show_param=off
      settings: xl_area=[0, 0, 0, 0, 0, 0, 0]
  barrel_switcher : Subsystem
      settings: AttributesFormatString=n_inputs=2
  bram_rd_addrs : xbsIndex_r3/Slice  mode=Lower Bit Location + Width  nbits=11  bit1=0  base1=MSB of Input  bit0=2  base0=LSB of Input  boolean_output=off  explicit_period=off  period=1  dbl_ovrd=off
  bs_sel : xbsIndex_r3/Slice  mode=Lower Bit Location + Width  nbits=2  bit1=0  base1=MSB of Input  bit0=0  base0=LSB of Input  boolean_output=off  explicit_period=off  period=1  dbl_ovrd=off
  delay_dp : Subsystem  mask{ram_bits=11, bram_latency=4}
      mask prompts: ram_bits "Max Delay (2^?)"; bram_latency "BRAM Latency"
  delay_dp1 : Subsystem  mask{ram_bits=11, bram_latency=4}
      mask prompts: ram_bits "Max Delay (2^?)"; bram_latency "BRAM Latency"
  delay_dp2 : Subsystem  mask{ram_bits=11, bram_latency=4}
      mask prompts: ram_bits "Max Delay (2^?)"; bram_latency "BRAM Latency"
  delay_dp3 : Subsystem  mask{ram_bits=11, bram_latency=4}
      mask prompts: ram_bits "Max Delay (2^?)"; bram_latency "BRAM Latency"
  max_delay : xbsIndex_r3/Constant  const=8192  equ=P=C  arith_type=Unsigned  n_bits=32  bin_pt=0  opselect=C  inp2=PCIN>>17  opr=+  inp1=P  carry=CIN  iostate=0  explicit_period=on  period=1  dbl_ovrd=off
  max_delay_chk : xbsIndex_r3/Relational  mode=a<=b  latency=1  explicit_period=off  period=1  en=off  dbl_ovrd=off  show_param=off
      settings: xl_area=[0, 0, 0, 0, 0, 0, 0]
  mux_delay : xbsIndex_r3/Mux  inputs=2  precision=Full  arith_type="Signed  (2's comp)"  n_bits=8  bin_pt=2  quantization=Truncate  overflow=Wrap  latency=0  explicit_period=off  period=1  en=off  dbl_ovrd=off  show_param=off  mux_type=off  use_rpm=off  gen_core=off
      settings: xl_area=[0, 0, 0, 0, 0, 0, 0]
  sync_delay : Subsystem  mask(sync_delay){DelayLen=5}
      mask prompts: DelayLen "Delay Length:"
      mask help: Delay an infrequent boolean pulse by the specified number of clocks.
      mask init:
      | BitWidth = max(2, ceil(log2(DelayLen+1)));
      | UseCounter = 1;
      | if DelayLen == 0,
      | 	UseCounter = 0;
      | end
      mask Help: eval('xlWeb([getenv(''MLIB_ROOT''), ''\casper_library\doc\sync_delay_usage.html''])')
      mask Display: fprintf('Z^-%d', DelayLen)
  sync_out : Outport
  data_out1 : Outport  Port=2
  data_out2 : Outport  Port=3
  data_out3 : Outport  Port=4
  data_out4 : Outport  Port=5
  wires:
  max_delay/1 -> max_delay_chk/2, mux_delay/2
  max_delay_chk/1 -> mux_delay/1
  sync/1 -> sync_delay/1(In), Register/2
  data_in1/1 -> delay_dp/1(din)
  bram_rd_addrs/1 -> delay_dp/2(delay), AddSub1/1, AddSub2/1, AddSub3/1
  mux_delay/1 -> bram_rd_addrs/1, bs_sel/1
  bs_sel/1 -> Relational1/1, Relational2/1, Relational3/1, Delay/1
  Constant1/1 -> Relational1/2
  Relational1/1 -> Convert1/1
  Convert1/1 -> AddSub1/2
  barrel_switcher/2(Out1) -> data_out4/1
  AddSub1/1 -> delay_dp1/2(delay)
  data_in2/1 -> delay_dp1/1(din)
  delay_dp1/1(dout) -> barrel_switcher/5(In3)
  Constant2/1 -> Relational2/2
  Relational2/1 -> Convert2/1
  Convert2/1 -> AddSub2/2
  barrel_switcher/3(Out2) -> data_out3/1
  AddSub2/1 -> delay_dp2/2(delay)
  data_in3/1 -> delay_dp2/1(din)
  delay_dp2/1(dout) -> barrel_switcher/4(In2)
  Constant3/1 -> Relational3/2
  Relational3/1 -> Convert3/1
  Convert3/1 -> AddSub3/2
  barrel_switcher/4(Out3) -> data_out2/1
  AddSub3/1 -> delay_dp3/2(delay)
  data_in4/1 -> delay_dp3/1(din)
  delay_dp3/1(dout) -> barrel_switcher/3(In1)
  barrel_switcher/1(sync_out) -> sync_out/1
  barrel_switcher/5(Out4) -> data_out1/1
  sync_delay/1(Out) -> barrel_switcher/2(sync_in)
  delay_dp/1(dout) -> barrel_switcher/6(In4)
  Register/1 -> mux_delay/3, max_delay_chk/1
  delay/1 -> Register/1
  Delay/1 -> barrel_switcher/1(sel)

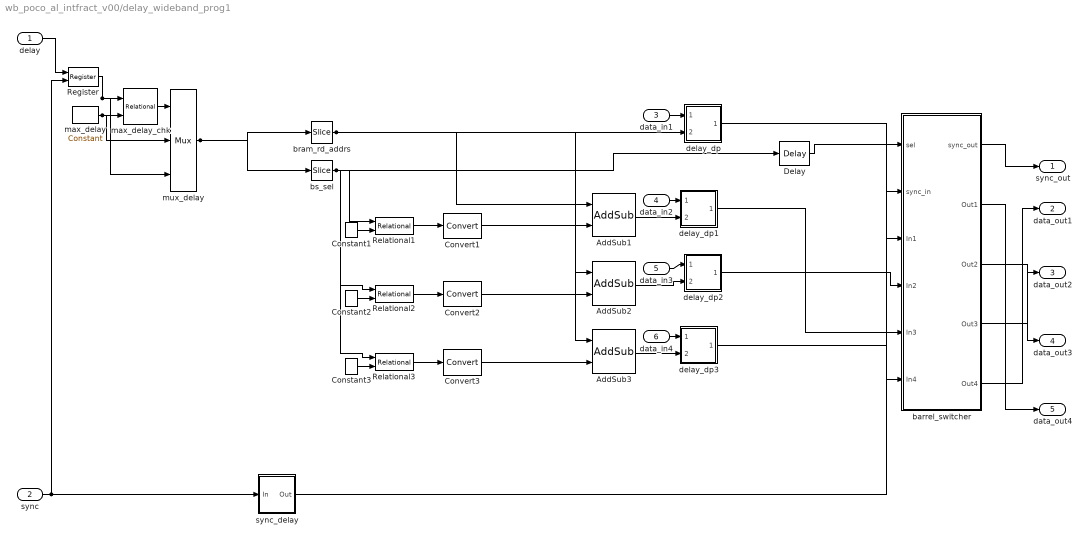
== system wb_poco_al_intfract_v00/delay_wideband_prog1 ==
  delay : Inport  Port=1  LatchInput=off
  sync : Inport  Port=2  LatchInput=off
  data_in1 : Inport  Port=3  LatchInput=off
  data_in2 : Inport  Port=4  LatchInput=off
  data_in3 : Inport  Port=5  LatchInput=off
  data_in4 : Inport  Port=6  LatchInput=off
  AddSub1 : xbsIndex_r3/AddSub  mode=Addition  precision=Full  arith_type=Unsigned  n_bits=11  bin_pt=0  quantization=Truncate  overflow=Wrap  latency=0  explicit_period=off  period=1  use_carryin=off  use_carryout=off  en=off  dbl_ovrd=off  show_param=off  use_core=on  pipeline=off  use_rpm=on  gen_core=off
      settings: xl_area=[0, 0, 0, 0, 0, 0, 0]
  AddSub2 : xbsIndex_r3/AddSub  mode=Addition  precision=Full  arith_type=Unsigned  n_bits=11  bin_pt=0  quantization=Truncate  overflow=Wrap  latency=0  explicit_period=off  period=1  use_carryin=off  use_carryout=off  en=off  dbl_ovrd=off  show_param=off  use_core=on  pipeline=off  use_rpm=on  gen_core=off
      settings: xl_area=[0, 0, 0, 0, 0, 0, 0]
  AddSub3 : xbsIndex_r3/AddSub  mode=Addition  precision=Full  arith_type=Unsigned  n_bits=11  bin_pt=0  quantization=Truncate  overflow=Wrap  latency=0  explicit_period=off  period=1  use_carryin=off  use_carryout=off  en=off  dbl_ovrd=off  show_param=off  use_core=on  pipeline=off  use_rpm=on  gen_core=off
      settings: xl_area=[0, 0, 0, 0, 0, 0, 0]
  Constant1 : xbsIndex_r3/Constant  const=2  equ=P=C  arith_type=Unsigned  n_bits=2  bin_pt=0  opselect=C  inp2=PCIN>>17  opr=+  inp1=P  carry=CIN  iostate=0  explicit_period=on  period=1  dbl_ovrd=off
  Constant2 : xbsIndex_r3/Constant  const=1  equ=P=C  arith_type=Unsigned  n_bits=2  bin_pt=0  opselect=C  inp2=PCIN>>17  opr=+  inp1=P  carry=CIN  iostate=0  explicit_period=on  period=1  dbl_ovrd=off
  Constant3 : xbsIndex_r3/Constant  const=0  equ=P=C  arith_type=Unsigned  n_bits=2  bin_pt=0  opselect=C  inp2=PCIN>>17  opr=+  inp1=P  carry=CIN  iostate=0  explicit_period=on  period=1  dbl_ovrd=off
  Convert1 : xbsIndex_r3/Convert  arith_type=Unsigned  n_bits=1  bin_pt=0  quantization=Truncate  overflow=Wrap  latency=0  explicit_period=off  period=1  dbl_ovrd=off  show_param=off  inserted_by_tool=off  pipeline=off
      settings: xl_area=[0, 0, 0, 0, 0, 0, 0]
  Convert2 : xbsIndex_r3/Convert  arith_type=Unsigned  n_bits=1  bin_pt=0  quantization=Truncate  overflow=Wrap  latency=0  explicit_period=off  period=1  dbl_ovrd=off  show_param=off  inserted_by_tool=off  pipeline=off
      settings: xl_area=[0, 0, 0, 0, 0, 0, 0]
  Convert3 : xbsIndex_r3/Convert  arith_type=Unsigned  n_bits=1  bin_pt=0  quantization=Truncate  overflow=Wrap  latency=0  explicit_period=off  period=1  dbl_ovrd=off  show_param=off  inserted_by_tool=off  pipeline=off
      settings: xl_area=[0, 0, 0, 0, 0, 0, 0]
  Delay : xbsIndex_r3/Delay  latency=5  reg_retiming=off  explicit_period=off  period=1  en=off  accept_only_valid=off  init_zero=on  dbl_ovrd=off  show_param=off
      settings: xl_area=[0, 0, 0, 0, 0, 0, 0]
  Register : xbsIndex_r3/Register  init=0  reg_only_valid=off  explicit_period=off  period=1  rst=off  en=on  out_en=off  dbl_ovrd=off  show_param=off
      settings: xl_area=[0, 0, 0, 0, 0, 0, 0]
  Relational1 : xbsIndex_r3/Relational  mode=a>b  latency=0  explicit_period=off  period=1  en=off  dbl_ovrd=off  show_param=off
      settings: xl_area=[0, 0, 0, 0, 0, 0, 0]
  Relational2 : xbsIndex_r3/Relational  mode=a>b  latency=0  explicit_period=off  period=1  en=off  dbl_ovrd=off  show_param=off
      settings: xl_area=[0, 0, 0, 0, 0, 0, 0]
  Relational3 : xbsIndex_r3/Relational  mode=a>b  latency=0  explicit_period=off  period=1  en=off  dbl_ovrd=off  show_param=off
      settings: xl_area=[0, 0, 0, 0, 0, 0, 0]
  barrel_switcher : Subsystem
      settings: AttributesFormatString=n_inputs=2
  bram_rd_addrs : xbsIndex_r3/Slice  mode=Lower Bit Location + Width  nbits=11  bit1=0  base1=MSB of Input  bit0=2  base0=LSB of Input  boolean_output=off  explicit_period=off  period=1  dbl_ovrd=off
  bs_sel : xbsIndex_r3/Slice  mode=Lower Bit Location + Width  nbits=2  bit1=0  base1=MSB of Input  bit0=0  base0=LSB of Input  boolean_output=off  explicit_period=off  period=1  dbl_ovrd=off
  delay_dp : Subsystem  mask{ram_bits=11, bram_latency=4}
      mask prompts: ram_bits "Max Delay (2^?)"; bram_latency "BRAM Latency"
  delay_dp1 : Subsystem  mask{ram_bits=11, bram_latency=4}
      mask prompts: ram_bits "Max Delay (2^?)"; bram_latency "BRAM Latency"
  delay_dp2 : Subsystem  mask{ram_bits=11, bram_latency=4}
      mask prompts: ram_bits "Max Delay (2^?)"; bram_latency "BRAM Latency"
  delay_dp3 : Subsystem  mask{ram_bits=11, bram_latency=4}
      mask prompts: ram_bits "Max Delay (2^?)"; bram_latency "BRAM Latency"
  max_delay : xbsIndex_r3/Constant  const=8192  equ=P=C  arith_type=Unsigned  n_bits=32  bin_pt=0  opselect=C  inp2=PCIN>>17  opr=+  inp1=P  carry=CIN  iostate=0  explicit_period=on  period=1  dbl_ovrd=off
  max_delay_chk : xbsIndex_r3/Relational  mode=a<=b  latency=1  explicit_period=off  period=1  en=off  dbl_ovrd=off  show_param=off
      settings: xl_area=[0, 0, 0, 0, 0, 0, 0]
  mux_delay : xbsIndex_r3/Mux  inputs=2  precision=Full  arith_type="Signed  (2's comp)"  n_bits=8  bin_pt=2  quantization=Truncate  overflow=Wrap  latency=0  explicit_period=off  period=1  en=off  dbl_ovrd=off  show_param=off  mux_type=off  use_rpm=off  gen_core=off
      settings: xl_area=[0, 0, 0, 0, 0, 0, 0]
  sync_delay : Subsystem  mask(sync_delay){DelayLen=5}
      mask prompts: DelayLen "Delay Length:"
      mask help: Delay an infrequent boolean pulse by the specified number of clocks.
      mask init:
      | BitWidth = max(2, ceil(log2(DelayLen+1)));
      | UseCounter = 1;
      | if DelayLen == 0,
      | 	UseCounter = 0;
      | end
      mask Help: eval('xlWeb([getenv(''MLIB_ROOT''), ''\casper_library\doc\sync_delay_usage.html''])')
      mask Display: fprintf('Z^-%d', DelayLen)
  sync_out : Outport
  data_out1 : Outport  Port=2
  data_out2 : Outport  Port=3
  data_out3 : Outport  Port=4
  data_out4 : Outport  Port=5
  wires:
  Delay/1 -> barrel_switcher/1(sel)
  delay/1 -> Register/1
  Register/1 -> max_delay_chk/1, mux_delay/3
  delay_dp/1(dout) -> barrel_switcher/6(In4)
  sync_delay/1(Out) -> barrel_switcher/2(sync_in)
  barrel_switcher/5(Out4) -> data_out1/1
  barrel_switcher/1(sync_out) -> sync_out/1
  delay_dp3/1(dout) -> barrel_switcher/3(In1)
  data_in4/1 -> delay_dp3/1(din)
  AddSub3/1 -> delay_dp3/2(delay)
  barrel_switcher/4(Out3) -> data_out2/1
  Convert3/1 -> AddSub3/2
  Relational3/1 -> Convert3/1
  Constant3/1 -> Relational3/2
  delay_dp2/1(dout) -> barrel_switcher/4(In2)
  data_in3/1 -> delay_dp2/1(din)
  AddSub2/1 -> delay_dp2/2(delay)
  barrel_switcher/3(Out2) -> data_out3/1
  Convert2/1 -> AddSub2/2
  Relational2/1 -> Convert2/1
  Constant2/1 -> Relational2/2
  delay_dp1/1(dout) -> barrel_switcher/5(In3)
  data_in2/1 -> delay_dp1/1(din)
  AddSub1/1 -> delay_dp1/2(delay)
  barrel_switcher/2(Out1) -> data_out4/1
  Convert1/1 -> AddSub1/2
  Relational1/1 -> Convert1/1
  Constant1/1 -> Relational1/2
  bs_sel/1 -> Delay/1, Relational3/1, Relational2/1, Relational1/1
  mux_delay/1 -> bs_sel/1, bram_rd_addrs/1
  bram_rd_addrs/1 -> AddSub3/1, AddSub2/1, AddSub1/1, delay_dp/2(delay)
  data_in1/1 -> delay_dp/1(din)
  sync/1 -> Register/2, sync_delay/1(In)
  max_delay_chk/1 -> mux_delay/1
  max_delay/1 -> mux_delay/2, max_delay_chk/2

== system wb_poco_al_intfract_v00/dir_x ==
  new_acc : Inport  Port=1  LatchInput=off
  a : Inport  Port=2  LatchInput=off
  b : Inport  Port=3  LatchInput=off
  c : Inport  Port=4  LatchInput=off
  d : Inport  Port=5  LatchInput=off
  aa : Subsystem  mask{n_chans=n_chans}
      mask prompts: n_chans "Number of channels"
      mask init:
      | chan_bits=ceil(log2(n_chans))
  ac : Subsystem  mask{n_chans=n_chans}
      mask prompts: n_chans "Number of Channels"
      mask init:
      | chan_bits=ceil(log2(n_chans))
  bb : Subsystem  mask{n_chans=n_chans}
      mask prompts: n_chans "Number of channels"
      mask init:
      | chan_bits=ceil(log2(n_chans))
  bd : Subsystem  mask{n_chans=n_chans}
      mask prompts: n_chans "Number of Channels"
      mask init:
      | chan_bits=ceil(log2(n_chans))
  cc : Subsystem  mask{n_chans=n_chans}
      mask prompts: n_chans "Number of channels"
      mask init:
      | chan_bits=ceil(log2(n_chans))
  dd : Subsystem  mask{n_chans=n_chans}
      mask prompts: n_chans "Number of channels"
      mask init:
      | chan_bits=ceil(log2(n_chans))
  wires:
  a/1 -> aa/2(c+di), aa/1(a+bi), ac/1(a+bi)
  new_acc/1 -> cc/3(new_acc), ac/3(new_acc), dd/3(new_acc), bd/3(new_acc), bb/3(new_acc), aa/3(new_acc)
  c/1 -> ac/2(c+di), cc/1(a+bi), cc/2(c+di)
  d/1 -> bd/2(c+di), dd/2(c+di), dd/1(a+bi)
  b/1 -> bb/1(a+bi), bb/2(c+di), bd/1(a+bi)

== system wb_poco_al_intfract_v00/downshift1 ==
  din : Inport  Port=1  LatchInput=off
  Convert2 : xbsIndex_r3/Convert  arith_type="Signed  (2's comp)"  n_bits=18  bin_pt=15  quantization="Round  (unbiased: Even Values)"  overflow=Wrap  latency=2  explicit_period=off  period=1  dbl_ovrd=off  show_param=off  inserted_by_tool=off  pipeline=off
      settings: xl_area=[0, 0, 0, 0, 0, 0, 0]
  Reinterpret : xbsIndex_r3/Reinterpret  force_arith_type=on  arith_type="Signed  (2's comp)"  force_bin_pt=on  bin_pt=17  force_valid=on
  Reinterpret3 : xbsIndex_r3/Reinterpret  force_arith_type=on  arith_type=Unsigned  force_bin_pt=on  bin_pt=0  force_valid=on
  Slice2 : xbsIndex_r3/Slice  mode=Upper Bit Location + Width  nbits=18  bit1=0  base1=MSB of Input  bit0=0  base0=LSB of Input  boolean_output=off  explicit_period=off  period=1  dbl_ovrd=off
  dout : Outport
  wires:
  Slice2/1 -> Reinterpret/1
  din/1 -> Slice2/1
  Reinterpret3/1 -> dout/1
  Reinterpret/1 -> Convert2/1
  Convert2/1 -> Reinterpret3/1

== system wb_poco_al_intfract_v00/downshift2 ==
  din : Inport  Port=1  LatchInput=off
  Convert2 : xbsIndex_r3/Convert  arith_type="Signed  (2's comp)"  n_bits=18  bin_pt=15  quantization="Round  (unbiased: Even Values)"  overflow=Wrap  latency=2  explicit_period=off  period=1  dbl_ovrd=off  show_param=off  inserted_by_tool=off  pipeline=off
      settings: xl_area=[0, 0, 0, 0, 0, 0, 0]
  Reinterpret : xbsIndex_r3/Reinterpret  force_arith_type=on  arith_type="Signed  (2's comp)"  force_bin_pt=on  bin_pt=17  force_valid=on
  Reinterpret3 : xbsIndex_r3/Reinterpret  force_arith_type=on  arith_type=Unsigned  force_bin_pt=on  bin_pt=0  force_valid=on
  Slice2 : xbsIndex_r3/Slice  mode=Upper Bit Location + Width  nbits=18  bit1=0  base1=MSB of Input  bit0=0  base0=LSB of Input  boolean_output=off  explicit_period=off  period=1  dbl_ovrd=off
  dout : Outport
  wires:
  Convert2/1 -> Reinterpret3/1
  Reinterpret/1 -> Convert2/1
  Reinterpret3/1 -> dout/1
  din/1 -> Slice2/1
  Slice2/1 -> Reinterpret/1

== system wb_poco_al_intfract_v00/downshift3 ==
  din : Inport  Port=1  LatchInput=off
  Convert2 : xbsIndex_r3/Convert  arith_type="Signed  (2's comp)"  n_bits=18  bin_pt=15  quantization="Round  (unbiased: Even Values)"  overflow=Wrap  latency=2  explicit_period=off  period=1  dbl_ovrd=off  show_param=off  inserted_by_tool=off  pipeline=off
      settings: xl_area=[0, 0, 0, 0, 0, 0, 0]
  Reinterpret : xbsIndex_r3/Reinterpret  force_arith_type=on  arith_type="Signed  (2's comp)"  force_bin_pt=on  bin_pt=17  force_valid=on
  Reinterpret3 : xbsIndex_r3/Reinterpret  force_arith_type=on  arith_type=Unsigned  force_bin_pt=on  bin_pt=0  force_valid=on
  Slice2 : xbsIndex_r3/Slice  mode=Upper Bit Location + Width  nbits=18  bit1=0  base1=MSB of Input  bit0=0  base0=LSB of Input  boolean_output=off  explicit_period=off  period=1  dbl_ovrd=off
  dout : Outport
  wires:
  Convert2/1 -> Reinterpret3/1
  Reinterpret/1 -> Convert2/1
  Reinterpret3/1 -> dout/1
  din/1 -> Slice2/1
  Slice2/1 -> Reinterpret/1

== system wb_poco_al_intfract_v00/downshift4 ==
  din : Inport  Port=1  LatchInput=off
  Convert2 : xbsIndex_r3/Convert  arith_type="Signed  (2's comp)"  n_bits=18  bin_pt=15  quantization="Round  (unbiased: Even Values)"  overflow=Wrap  latency=2  explicit_period=off  period=1  dbl_ovrd=off  show_param=off  inserted_by_tool=off  pipeline=off
      settings: xl_area=[0, 0, 0, 0, 0, 0, 0]
  Reinterpret : xbsIndex_r3/Reinterpret  force_arith_type=on  arith_type="Signed  (2's comp)"  force_bin_pt=on  bin_pt=17  force_valid=on
  Reinterpret3 : xbsIndex_r3/Reinterpret  force_arith_type=on  arith_type=Unsigned  force_bin_pt=on  bin_pt=0  force_valid=on
  Slice2 : xbsIndex_r3/Slice  mode=Upper Bit Location + Width  nbits=18  bit1=0  base1=MSB of Input  bit0=0  base0=LSB of Input  boolean_output=off  explicit_period=off  period=1  dbl_ovrd=off
  dout : Outport
  wires:
  Slice2/1 -> Reinterpret/1
  din/1 -> Slice2/1
  Reinterpret3/1 -> dout/1
  Reinterpret/1 -> Convert2/1
  Convert2/1 -> Reinterpret3/1

== system wb_poco_al_intfract_v00/downshift5 ==
  din : Inport  Port=1  LatchInput=off
  Convert2 : xbsIndex_r3/Convert  arith_type="Signed  (2's comp)"  n_bits=18  bin_pt=15  quantization="Round  (unbiased: Even Values)"  overflow=Wrap  latency=2  explicit_period=off  period=1  dbl_ovrd=off  show_param=off  inserted_by_tool=off  pipeline=off
      settings: xl_area=[0, 0, 0, 0, 0, 0, 0]
  Reinterpret : xbsIndex_r3/Reinterpret  force_arith_type=on  arith_type="Signed  (2's comp)"  force_bin_pt=on  bin_pt=17  force_valid=on
  Reinterpret3 : xbsIndex_r3/Reinterpret  force_arith_type=on  arith_type=Unsigned  force_bin_pt=on  bin_pt=0  force_valid=on
  Slice2 : xbsIndex_r3/Slice  mode=Upper Bit Location + Width  nbits=18  bit1=0  base1=MSB of Input  bit0=0  base0=LSB of Input  boolean_output=off  explicit_period=off  period=1  dbl_ovrd=off
  dout : Outport
  wires:
  Convert2/1 -> Reinterpret3/1
  Reinterpret/1 -> Convert2/1
  Reinterpret3/1 -> dout/1
  din/1 -> Slice2/1
  Slice2/1 -> Reinterpret/1

== system wb_poco_al_intfract_v00/downshift6 ==
  din : Inport  Port=1  LatchInput=off
  Convert2 : xbsIndex_r3/Convert  arith_type="Signed  (2's comp)"  n_bits=18  bin_pt=15  quantization="Round  (unbiased: Even Values)"  overflow=Wrap  latency=2  explicit_period=off  period=1  dbl_ovrd=off  show_param=off  inserted_by_tool=off  pipeline=off
      settings: xl_area=[0, 0, 0, 0, 0, 0, 0]
  Reinterpret : xbsIndex_r3/Reinterpret  force_arith_type=on  arith_type="Signed  (2's comp)"  force_bin_pt=on  bin_pt=17  force_valid=on
  Reinterpret3 : xbsIndex_r3/Reinterpret  force_arith_type=on  arith_type=Unsigned  force_bin_pt=on  bin_pt=0  force_valid=on
  Slice2 : xbsIndex_r3/Slice  mode=Upper Bit Location + Width  nbits=18  bit1=0  base1=MSB of Input  bit0=0  base0=LSB of Input  boolean_output=off  explicit_period=off  period=1  dbl_ovrd=off
  dout : Outport
  wires:
  Slice2/1 -> Reinterpret/1
  din/1 -> Slice2/1
  Reinterpret3/1 -> dout/1
  Reinterpret/1 -> Convert2/1
  Convert2/1 -> Reinterpret3/1

== system wb_poco_al_intfract_v00/downshift7 ==
  din : Inport  Port=1  LatchInput=off
  Convert2 : xbsIndex_r3/Convert  arith_type="Signed  (2's comp)"  n_bits=18  bin_pt=15  quantization="Round  (unbiased: Even Values)"  overflow=Wrap  latency=2  explicit_period=off  period=1  dbl_ovrd=off  show_param=off  inserted_by_tool=off  pipeline=off
      settings: xl_area=[0, 0, 0, 0, 0, 0, 0]
  Reinterpret : xbsIndex_r3/Reinterpret  force_arith_type=on  arith_type="Signed  (2's comp)"  force_bin_pt=on  bin_pt=17  force_valid=on
  Reinterpret3 : xbsIndex_r3/Reinterpret  force_arith_type=on  arith_type=Unsigned  force_bin_pt=on  bin_pt=0  force_valid=on
  Slice2 : xbsIndex_r3/Slice  mode=Upper Bit Location + Width  nbits=18  bit1=0  base1=MSB of Input  bit0=0  base0=LSB of Input  boolean_output=off  explicit_period=off  period=1  dbl_ovrd=off
  dout : Outport
  wires:
  Slice2/1 -> Reinterpret/1
  din/1 -> Slice2/1
  Reinterpret3/1 -> dout/1
  Reinterpret/1 -> Convert2/1
  Convert2/1 -> Reinterpret3/1
